simulink model "DT_MotorCC_Multibody_wo_vib"  (R2023b)
settings: Solver=FixedStepAuto  StartTime=0.0  StopTime=5  FixedStep=0.001  RelTol=1e-3
model workspace (MAT data in the model file):
  A = 5
  Frec = 1
  a = 1
values from neighbouring files (symbols this model uses):
  J = (tau_m * K^2)/(Ra)    (= 0.000330907721143)    [Parameters_MotorCC.m]
  K_reductora = 1/30    (= 0.0333333333333)    [Parameters_MotorCC.m]
  K_taco = 8.07e-3    (= 0.00807)    [Parameters_MotorCC.m]
  PWM_sat = 8.78    [Parameters_MotorCC.m]
  ZM_pot = 17.5    [Parameters_MotorCC.m]
undefined symbols (not defined in the file or in its folder): smiData, X, Y, Z
libraries: fl_lib x37, nesl_utility x26, sm_lib x16, ee_lib x7, simulink x2, slpidlib x2, sdl_lib x1
(part 2 of 2)

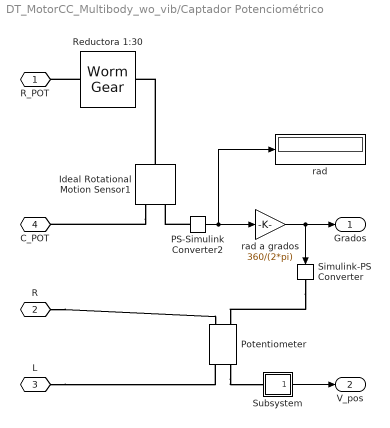
== system DT_MotorCC_Multibody_wo_vib/Captador Potenciométrico ==
  Ideal Rotational Motion Sensor1 : fl_lib/Mechanical/Mechanical Sensors/Ideal Rotational Motion Sensor  reference=foundation.enum.MeasurementReference.difference  acceleration_port=false  velocity_port=false  position_port=true  wrap_angle=true  offset=0 rad
      settings: InternalSimscapePortConfiguration="{\"Bottom\":[],\"Left\":[{\"id\":\"R\",\"label\":\"R\",\"type\":\"foundation.mechanical.rotational.rotational\"}],\"Right\":[{\"id\":\"C\",\"label\":\"C\",\"type\":\"foundation.mechanical.rotational.rotational\"},{\"id\":\"A\",\"label\":\"A\",\"type\":\"output\"}],\"Top\":[]}"
  PS-Simulink Converter2 : nesl_utility/PS-Simulink Converter  PhysicalDomain=network_engine_domain  SubClassName=ps_output  LeftPortType=input  RightPortType=output  PseudoPeriodic=off  Frequencies=[]  VectorFormat=inherit  Unit=rad  AffineConversion=off
  Potentiometer : ee_lib/Passive/Potentiometer  nPorts=ee.enum.passive.potentiometer.nPorts.Three  R0=9.77 kOhm  Rw=1 Ohm  xmin=0  xmax=360-ZM_pot  minResistance=1 Ohm  maxResistance=9999 Ohm  xmin2port=0  xmax2port=360  Taper=ee.enum.passive.potentiometer.linOrLog.lin  Rcenter=200 Ohm  Gradient=ee.enum.passive.potentiometer.gradient.higherR
      settings: InternalSimscapePortConfiguration="{\"Bottom\":[],\"Left\":[{\"id\":\"pinL\",\"label\":\"L\",\"type\":\"foundation.electrical.electrical\"},{\"id\":\"W\",\"label\":\"W\",\"type\":\"foundation.electrical.electrical\"}],\"Right\":[{\"id\":\"pinR\",\"label\":\"R\",\"type\":\"foundation.electrical.electrical\"},{\"id\":\"x\",\"label\":\"x\",\"type\":\"input\"}],\"Top\":[]}"
  Reductora 1:30 : sdl_lib/Gears/Worm Gear  ratio=1/K_reductora  thread_type=sdl.enum.handedness.right  friction_model=sdl.enum.gear_friction.none  friction_parameterization=sdl.enum.efficiency_geometry.geometry  pr_ang=17.5 deg  lead_ang=20 deg  fr_coeff=0.08  eff_wg=0.74  eff_gw=0.65  temperature_TLU=[280, 300, 320] K  efficiency_wg_TLU=[.75, .65, .6]  efficiency_gw_TLU=[.5, .45, .4]  pwr_thr=0.001 W  mu_visc=[0, 0] N*m*s/rad  thermal_mass=50 J/K  temperature_specify=off  temperature_priority=High  temperature=300 K  temperature_nominal_specify=off  temperature_nominal_unit=K  temperature_nominal_value=1
      settings: InternalSimscapePortConfiguration="{\"Bottom\":[],\"Left\":[{\"id\":\"W\",\"label\":\"W\",\"type\":\"foundation.mechanical.rotational.rotational\"}],\"Right\":[{\"id\":\"G\",\"label\":\"G\",\"type\":\"foundation.mechanical.rotational.rotational\"}],\"Top\":[]}"
  Simulink-PS Converter : nesl_utility/Simulink-PS Converter  PhysicalDomain=network_engine_domain  SubClassName=ps_input  LeftPortType=input  RightPortType=output  PseudoPeriodic=off  Frequencies=[]  NoiseDistribution=none  NoiseParameters=[]  Unit=1  AffineConversion=off  FilteringAndDerivatives=provide  SimscapeFilterOrder=1  InputFilterTimeConstant=0.001  UdotUserProvided=0
  Subsystem : Subsystem
      mask Display: disp('V');
  rad : Display
  rad a grados : Gain  Gain=360/(2*pi)
  R_POT : PMIOPort  Side=Left
  R : PMIOPort  Port=2  Side=Left
  L : PMIOPort  Port=3  Side=Left
  C_POT : PMIOPort  Port=4  Side=Left
  Grados : Outport
  V_pos : Outport  Port=2
  wires:
  rad a grados/1 -> Grados/1, Simulink-PS Converter/1
  PS-Simulink Converter2/1 -> rad/1, rad a grados/1
  Subsystem/1(output) -> V_pos/1
  connections:
  Ideal Rotational Motion Sensor1/RConn1 -- C_POT/RConn1
  PS-Simulink Converter2/LConn1 -- Ideal Rotational Motion Sensor1/RConn2
  Ideal Rotational Motion Sensor1/LConn1 -- Reductora 1:30/RConn1
  L/RConn1 -- Potentiometer/LConn1
  R/RConn1 -- Potentiometer/RConn1
  Reductora 1:30/LConn1 -- R_POT/RConn1
  Potentiometer/LConn2 -- Subsystem/LConn1
  Simulink-PS Converter/RConn1 -- Potentiometer/RConn2

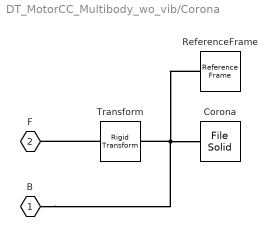
== system DT_MotorCC_Multibody_wo_vib/Corona ==
  Corona : sm_lib/Body Elements/File Solid  ExtGeomFileName=Eje_Corona.STEP  UnitType=FromFile  ExtGeomFileUnits=m  StepReaderType=HEX  ExportConvexHullGeometry=off  InertiaType=Custom  Mass=smiData.Solid(1).mass  MassUnits=kg  CenterOfMass=smiData.Solid(1).CoM  CenterOfMassUnits=mm  MomentsOfInertia=[0 0 0]  MomentsOfInertiaUnits=kg*mm^2  ProductsOfInertia=[0 0 0]  ProductsOfInertiaUnits=kg*mm^2  BasedOnType=DensityFromFile  Density=1000  DensityUnits=kg/m^3  DoExposeReferenceFrame=on  SerializedFrames=<Frames/>  GraphicType=FromGeometry  MarkerShape=Sphere  MarkerSize=10  GraphicVisPropType=SimpleVisualProperties  GraphicDiffuseColor=smiData.Solid(1).color  GraphicSpecularColor=[0.5 0.5 0.5 1.0]  GraphicAmbientColor=[0.15 0.15 0.15 1.0]  GraphicEmissiveColor=[0.0 0.0 0.0 1.0]  GraphicShininess=75  GraphicOpacity=smiData.Solid(1).opacity
  ReferenceFrame : sm_lib/Frames and Transforms/Reference Frame
  Transform : sm_lib/Frames and Transforms/Rigid Transform  TranslationMethod=Cartesian  TranslationStandardOffset=0  TranslationStandardOffsetUnits=m  TranslationStandardAxis=+Z  TranslationCartesianOffset=smiData.RigidTransform(4).translation  TranslationCartesianOffsetUnits=mm  TranslationROffset=0  TranslationROffsetUnits=m  TranslationZOffset=0  TranslationZOffsetUnits=m  TranslationThetaOffset=0  TranslationThetaOffsetUnits=deg  RotationMethod=ArbitraryAxis  RotationAngleUnits=rad  RotationStandardAxis=+Z  RotationAngle=smiData.RigidTransform(4).angle  RotationArbitraryAxis=smiData.RigidTransform(4).axis  FollAlignAxisA=+X  BaseAlignAxisA=+Y  FollAlignAxisB=+Y  BaseAlignAxisB=+Z  RotationSequenceAxes=FollowerAxes  RotationSequence=XYX  RotationSequenceAngles=[0 0 0]  RotationSequenceAnglesUnits=deg  RotationMatrix=[1 0 0; 0 1 0; 0 0 1]  Quaternion=[1 0 0 0]
  B : PMIOPort  Side=Left
  F : PMIOPort  Port=2  Side=Left
  connections:
  ReferenceFrame/RConn1 -- B/RConn1 -- Corona/RConn1 -- Transform/LConn1
  Transform/RConn1 -- F/RConn1

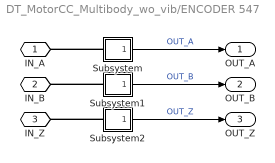
== system DT_MotorCC_Multibody_wo_vib/ENCODER 547 ==
  Subsystem : Subsystem
      mask Display: disp('V');
  Subsystem1 : Subsystem
      mask Display: disp('V');
  Subsystem2 : Subsystem
      mask Display: disp('V');
  IN_A : PMIOPort  Side=Left
  IN_B : PMIOPort  Port=2  Side=Left
  IN_Z : PMIOPort  Port=3  Side=Left
  OUT_A : Outport
  OUT_B : Outport  Port=2
  OUT_Z : Outport  Port=3
  wires:
  Subsystem2/1(output) -> OUT_Z/1  "OUT_Z"
  Subsystem1/1(output) -> OUT_B/1  "OUT_B"
  Subsystem/1(output) -> OUT_A/1  "OUT_A"
  connections:
  Subsystem/LConn1 -- IN_A/RConn1
  Subsystem1/LConn1 -- IN_B/RConn1
  Subsystem2/LConn1 -- IN_Z/RConn1

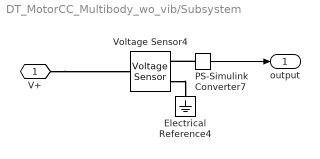
== system DT_MotorCC_Multibody_wo_vib/Subsystem ==
  Electrical Reference4 : fl_lib/Electrical/Electrical Elements/Electrical Reference
  PS-Simulink Converter7 : nesl_utility/PS-Simulink Converter  PhysicalDomain=network_engine_domain  SubClassName=ps_output  LeftPortType=input  RightPortType=output  PseudoPeriodic=off  Frequencies=[]  VectorFormat=inherit  Unit=V  AffineConversion=off
  Voltage Sensor4 : fl_lib/Electrical/Electrical Sensors/Voltage Sensor
  V+ : PMIOPort  Side=Left
  output : Outport
  wires:
  PS-Simulink Converter7/1 -> output/1
  connections:
  PS-Simulink Converter7/LConn1 -- Voltage Sensor4/RConn1
  Voltage Sensor4/RConn2 -- Electrical Reference4/LConn1
  V+/RConn1 -- Voltage Sensor4/LConn1

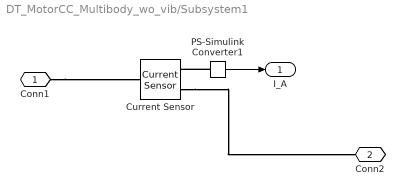
== system DT_MotorCC_Multibody_wo_vib/Subsystem1 ==
  Current Sensor : fl_lib/Electrical/Electrical Sensors/Current Sensor
  PS-Simulink Converter1 : nesl_utility/PS-Simulink Converter  PhysicalDomain=network_engine_domain  SubClassName=ps_output  LeftPortType=input  RightPortType=output  PseudoPeriodic=off  Frequencies=[]  VectorFormat=inherit  Unit=A  AffineConversion=off
  Conn1 : PMIOPort  Side=Left
  Conn2 : PMIOPort  Port=2  Side=Right
  I_A : Outport
  wires:
  PS-Simulink Converter1/1 -> I_A/1
  connections:
  PS-Simulink Converter1/LConn1 -- Current Sensor/RConn1
  Conn1/RConn1 -- Current Sensor/LConn1
  Current Sensor/RConn2 -- Conn2/RConn1

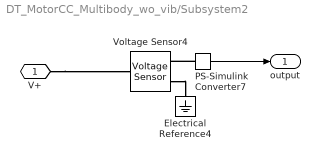
== system DT_MotorCC_Multibody_wo_vib/Subsystem2 ==
  Electrical Reference4 : fl_lib/Electrical/Electrical Elements/Electrical Reference
  PS-Simulink Converter7 : nesl_utility/PS-Simulink Converter  PhysicalDomain=network_engine_domain  SubClassName=ps_output  LeftPortType=input  RightPortType=output  PseudoPeriodic=off  Frequencies=[]  VectorFormat=inherit  Unit=V  AffineConversion=off
  Voltage Sensor4 : fl_lib/Electrical/Electrical Sensors/Voltage Sensor
  V+ : PMIOPort  Side=Left
  output : Outport
  wires:
  PS-Simulink Converter7/1 -> output/1
  connections:
  PS-Simulink Converter7/LConn1 -- Voltage Sensor4/RConn1
  Voltage Sensor4/RConn2 -- Electrical Reference4/LConn1
  V+/RConn1 -- Voltage Sensor4/LConn1

== system DT_MotorCC_Multibody_wo_vib/Subsystem3 ==
  Electrical Reference4 : fl_lib/Electrical/Electrical Elements/Electrical Reference
  PS-Simulink Converter7 : nesl_utility/PS-Simulink Converter  PhysicalDomain=network_engine_domain  SubClassName=ps_output  LeftPortType=input  RightPortType=output  PseudoPeriodic=off  Frequencies=[]  VectorFormat=inherit  Unit=V  AffineConversion=off
  Voltage Sensor4 : fl_lib/Electrical/Electrical Sensors/Voltage Sensor
  V+ : PMIOPort  Side=Left
  output : Outport
  wires:
  PS-Simulink Converter7/1 -> output/1
  connections:
  V+/RConn1 -- Voltage Sensor4/LConn1
  Voltage Sensor4/RConn2 -- Electrical Reference4/LConn1
  PS-Simulink Converter7/LConn1 -- Voltage Sensor4/RConn1

== system DT_MotorCC_Multibody_wo_vib/Subsystem4 ==
  Electrical Reference4 : fl_lib/Electrical/Electrical Elements/Electrical Reference
  PS-Simulink Converter7 : nesl_utility/PS-Simulink Converter  PhysicalDomain=network_engine_domain  SubClassName=ps_output  LeftPortType=input  RightPortType=output  PseudoPeriodic=off  Frequencies=[]  VectorFormat=inherit  Unit=V  AffineConversion=off
  Voltage Sensor4 : fl_lib/Electrical/Electrical Sensors/Voltage Sensor
  V+ : PMIOPort  Side=Left
  output : Outport
  wires:
  PS-Simulink Converter7/1 -> output/1
  connections:
  V+/RConn1 -- Voltage Sensor4/LConn1
  Voltage Sensor4/RConn2 -- Electrical Reference4/LConn1
  PS-Simulink Converter7/LConn1 -- Voltage Sensor4/RConn1

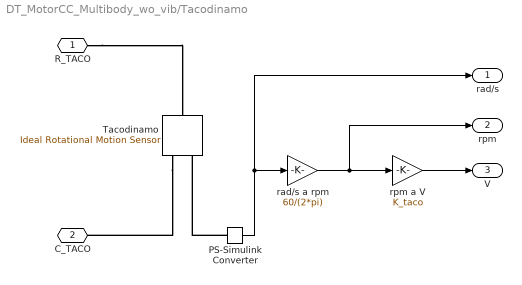
== system DT_MotorCC_Multibody_wo_vib/Tacodinamo ==
  PS-Simulink Converter : nesl_utility/PS-Simulink Converter  PhysicalDomain=network_engine_domain  SubClassName=ps_output  LeftPortType=input  RightPortType=output  PseudoPeriodic=off  Frequencies=[]  VectorFormat=inherit  Unit=rad/s  AffineConversion=off
  Tacodinamo : fl_lib/Mechanical/Mechanical Sensors/Ideal Rotational Motion Sensor  reference=foundation.enum.MeasurementReference.difference  acceleration_port=false  velocity_port=true  position_port=false  wrap_angle=true  offset=0 rad
      settings: InternalSimscapePortConfiguration="{\"Bottom\":[],\"Left\":[{\"id\":\"R\",\"label\":\"R\",\"type\":\"foundation.mechanical.rotational.rotational\"}],\"Right\":[{\"id\":\"C\",\"label\":\"C\",\"type\":\"foundation.mechanical.rotational.rotational\"},{\"id\":\"W\",\"label\":\"W\",\"type\":\"output\"}],\"Top\":[]}"
  rad/s a rpm : Gain  Gain=60/(2*pi)
  rpm a V : Gain  Gain=K_taco
  R_TACO : PMIOPort  Side=Left
  C_TACO : PMIOPort  Port=2  Side=Left
  rad/s : Outport
  rpm : Outport  Port=2
  V : Outport  Port=3
  wires:
  rpm a V/1 -> V/1
  rad/s a rpm/1 -> rpm/1, rpm a V/1
  PS-Simulink Converter/1 -> rad/s/1, rad/s a rpm/1
  connections:
  Tacodinamo/RConn1 -- C_TACO/RConn1
  PS-Simulink Converter/LConn1 -- Tacodinamo/RConn2
  R_TACO/RConn1 -- Tacodinamo/LConn1

== system DT_MotorCC_Multibody_wo_vib/Tornillo_sinfín ==
  ReferenceFrame : sm_lib/Frames and Transforms/Reference Frame
  Tornillo_sinfin : sm_lib/Body Elements/File Solid  ExtGeomFileName=Eje_Sinfin_Encoder.STEP  UnitType=FromFile  ExtGeomFileUnits=m  StepReaderType=HEX  ExportConvexHullGeometry=off  InertiaType=Custom  Mass=smiData.Solid(3).mass  MassUnits=kg  CenterOfMass=smiData.Solid(3).CoM  CenterOfMassUnits=mm  MomentsOfInertia=[0 0 0]  MomentsOfInertiaUnits=kg*mm^2  ProductsOfInertia=[0 0 0]  ProductsOfInertiaUnits=kg*mm^2  BasedOnType=Mass  Density=1000  DensityUnits=kg/m^3  DoExposeReferenceFrame=on  SerializedFrames=<Frames/>  GraphicType=FromGeometry  MarkerShape=Sphere  MarkerSize=10  GraphicVisPropType=SimpleVisualProperties  GraphicDiffuseColor=smiData.Solid(3).color  GraphicSpecularColor=[0.5 0.5 0.5 1.0]  GraphicAmbientColor=[0.15 0.15 0.15 1.0]  GraphicEmissiveColor=[0.0 0.0 0.0 1.0]  GraphicShininess=75  GraphicOpacity=smiData.Solid(3).opacity
  Transform : sm_lib/Frames and Transforms/Rigid Transform  TranslationMethod=Cartesian  TranslationStandardOffset=0  TranslationStandardOffsetUnits=m  TranslationStandardAxis=+Z  TranslationCartesianOffset=smiData.RigidTransform(2).translation  TranslationCartesianOffsetUnits=mm  TranslationROffset=0  TranslationROffsetUnits=m  TranslationZOffset=0  TranslationZOffsetUnits=m  TranslationThetaOffset=0  TranslationThetaOffsetUnits=deg  RotationMethod=ArbitraryAxis  RotationAngleUnits=rad  RotationStandardAxis=+Z  RotationAngle=smiData.RigidTransform(2).angle  RotationArbitraryAxis=smiData.RigidTransform(2).axis  FollAlignAxisA=+X  BaseAlignAxisA=+Y  FollAlignAxisB=+Y  BaseAlignAxisB=+Z  RotationSequenceAxes=FollowerAxes  RotationSequence=XYX  RotationSequenceAngles=[0 0 0]  RotationSequenceAnglesUnits=deg  RotationMatrix=[1 0 0; 0 1 0; 0 0 1]  Quaternion=[1 0 0 0]
  F : PMIOPort  Side=Left
  B : PMIOPort  Port=2  Side=Left
  connections:
  ReferenceFrame/RConn1 -- B/RConn1 -- Tornillo_sinfin/RConn1 -- Transform/LConn1
  Transform/RConn1 -- F/RConn1

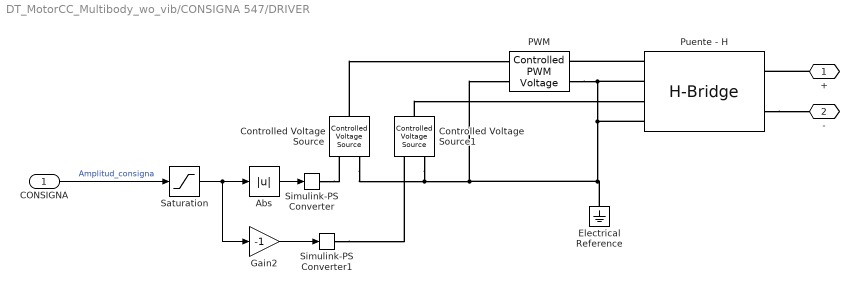
== system DT_MotorCC_Multibody_wo_vib/CONSIGNA 547/DRIVER ==
  CONSIGNA : Inport
  Abs : Abs  SaturateOnIntegerOverflow=off
  Controlled Voltage Source : fl_lib/Electrical/Electrical Sources/Controlled Voltage Source
  Controlled Voltage Source1 : fl_lib/Electrical/Electrical Sources/Controlled Voltage Source
  Electrical Reference : fl_lib/Electrical/Electrical Elements/Electrical Reference
  Gain2 : Gain  Gain=-1
  PWM : ee_lib/Integrated Circuits/Controlled PWM Voltage  F=PWM_freq kHz  TD=0 s  pulse_width_offset=0 s  pulse_min=0 s  pwm_or_av=ee.enum.pwm_or_av.averaged  event_type=ee.enum.ic.event.asynchronous  sample_time=1e-6 s  Vmin=0 V  Vmax=Input_100_Duty_Cycle V  Vm=PWM_out V  u_min=0  u_max=1
  Puente - H : ee_lib/Semiconductors & Converters/Converters/H-Bridge  supply_ports=ee.enum.supply_ports.hidesupply  pwm_or_av=ee.enum.pwm_or_av.averaged  regenerative_braking_mode=ee.enum.converters.regenerative_braking_mode.depends_on_rev  discontinuous=ee.enum.current_profile.continuous  freewheeling_mode=ee.enum.converters.freewheeling_mode.one_switch_one_diode  Rload=10 Ohm  Lload=1e-5 H  F=10 kHz  Venable=2.5 V  Vmax=PWM_out V  Vreverse=0.001 V  Vbrake=2.5 V  Vm=PWM_out V  Ron=0.1 Ohm  Don=0.05 Ohm  Goff=1e-6 S  Tmeas=298.15 K  Ron2=0.1 Ohm  Don2=0.05 Ohm  Tmeas2=398.15 K  thermal_mass=100 J/K  initial_temperature=298.15 K
  Saturation : Saturate  UpperLimit=PWM_sat  LowerLimit=-PWM_sat
  Simulink-PS Converter : nesl_utility/Simulink-PS Converter  PhysicalDomain=network_engine_domain  SubClassName=ps_input  LeftPortType=input  RightPortType=output  PseudoPeriodic=off  Frequencies=[]  NoiseDistribution=none  NoiseParameters=[]  Unit=1  AffineConversion=off  FilteringAndDerivatives=provide  SimscapeFilterOrder=1  InputFilterTimeConstant=0.001  UdotUserProvided=0
  Simulink-PS Converter1 : nesl_utility/Simulink-PS Converter  PhysicalDomain=network_engine_domain  SubClassName=ps_input  LeftPortType=input  RightPortType=output  PseudoPeriodic=off  Frequencies=[]  NoiseDistribution=none  NoiseParameters=[]  Unit=1  AffineConversion=off  FilteringAndDerivatives=provide  SimscapeFilterOrder=1  InputFilterTimeConstant=0.001  UdotUserProvided=0
  + : PMIOPort  Side=Right
  - : PMIOPort  Port=2  Side=Right
  wires:
  CONSIGNA/1 -> Saturation/1  "Amplitud_consigna"
  Abs/1 -> Simulink-PS Converter/1
  Gain2/1 -> Simulink-PS Converter1/1
  Saturation/1 -> Gain2/1, Abs/1
  connections:
  Puente - H/LConn1 -- PWM/RConn1
  Controlled Voltage Source/RConn2 -- PWM/LConn2 -- Electrical Reference/LConn1 -- Puente - H/LConn4 -- PWM/RConn2 -- Puente - H/LConn2 -- Controlled Voltage Source1/RConn2
  Controlled Voltage Source1/LConn1 -- Puente - H/LConn3
  Puente - H/RConn2 -- -/RConn1
  Controlled Voltage Source/LConn1 -- PWM/LConn1
  Simulink-PS Converter/RConn1 -- Controlled Voltage Source/RConn1
  Simulink-PS Converter1/RConn1 -- Controlled Voltage Source1/RConn1
  +/RConn1 -- Puente - H/RConn1

== system DT_MotorCC_Multibody_wo_vib/Captador Potenciométrico/Subsystem ==
  Electrical Reference4 : fl_lib/Electrical/Electrical Elements/Electrical Reference
  PS-Simulink Converter7 : nesl_utility/PS-Simulink Converter  PhysicalDomain=network_engine_domain  SubClassName=ps_output  LeftPortType=input  RightPortType=output  PseudoPeriodic=off  Frequencies=[]  VectorFormat=inherit  Unit=V  AffineConversion=off
  Voltage Sensor4 : fl_lib/Electrical/Electrical Sensors/Voltage Sensor
  V+ : PMIOPort  Side=Left
  output : Outport
  wires:
  PS-Simulink Converter7/1 -> output/1
  connections:
  PS-Simulink Converter7/LConn1 -- Voltage Sensor4/RConn1
  Voltage Sensor4/RConn2 -- Electrical Reference4/LConn1
  V+/RConn1 -- Voltage Sensor4/LConn1

== system DT_MotorCC_Multibody_wo_vib/ENCODER 547/Subsystem ==
  Electrical Reference4 : fl_lib/Electrical/Electrical Elements/Electrical Reference
  PS-Simulink Converter7 : nesl_utility/PS-Simulink Converter  PhysicalDomain=network_engine_domain  SubClassName=ps_output  LeftPortType=input  RightPortType=output  PseudoPeriodic=off  Frequencies=[]  VectorFormat=inherit  Unit=V  AffineConversion=off
  Voltage Sensor4 : fl_lib/Electrical/Electrical Sensors/Voltage Sensor
  V+ : PMIOPort  Side=Left
  output : Outport
  wires:
  PS-Simulink Converter7/1 -> output/1
  connections:
  PS-Simulink Converter7/LConn1 -- Voltage Sensor4/RConn1
  Voltage Sensor4/RConn2 -- Electrical Reference4/LConn1
  V+/RConn1 -- Voltage Sensor4/LConn1

== system DT_MotorCC_Multibody_wo_vib/ENCODER 547/Subsystem1 ==
  Electrical Reference4 : fl_lib/Electrical/Electrical Elements/Electrical Reference
  PS-Simulink Converter7 : nesl_utility/PS-Simulink Converter  PhysicalDomain=network_engine_domain  SubClassName=ps_output  LeftPortType=input  RightPortType=output  PseudoPeriodic=off  Frequencies=[]  VectorFormat=inherit  Unit=V  AffineConversion=off
  Voltage Sensor4 : fl_lib/Electrical/Electrical Sensors/Voltage Sensor
  V+ : PMIOPort  Side=Left
  output : Outport
  wires:
  PS-Simulink Converter7/1 -> output/1
  connections:
  PS-Simulink Converter7/LConn1 -- Voltage Sensor4/RConn1
  Voltage Sensor4/RConn2 -- Electrical Reference4/LConn1
  V+/RConn1 -- Voltage Sensor4/LConn1

== system DT_MotorCC_Multibody_wo_vib/ENCODER 547/Subsystem2 ==
  Electrical Reference4 : fl_lib/Electrical/Electrical Elements/Electrical Reference
  PS-Simulink Converter7 : nesl_utility/PS-Simulink Converter  PhysicalDomain=network_engine_domain  SubClassName=ps_output  LeftPortType=input  RightPortType=output  PseudoPeriodic=off  Frequencies=[]  VectorFormat=inherit  Unit=V  AffineConversion=off
  Voltage Sensor4 : fl_lib/Electrical/Electrical Sensors/Voltage Sensor
  V+ : PMIOPort  Side=Left
  output : Outport
  wires:
  PS-Simulink Converter7/1 -> output/1
  connections:
  PS-Simulink Converter7/LConn1 -- Voltage Sensor4/RConn1
  Voltage Sensor4/RConn2 -- Electrical Reference4/LConn1
  V+/RConn1 -- Voltage Sensor4/LConn1
